simulink model "BenchtopSkinpatch_SingleTone"  (R2016a)
settings: Solver=VariableStepAuto  StartTime=0.0  StopTime=sim_time  RelTol=1e-3
undefined symbols (not defined in the file): Fbit, Fs, Ts, Tsym
libraries: dspsigops x4, commdigbbndpm3 x1
settings Model: Creator=ckilfoyl  LastModifiedBy=ckilfoyl
settings DataIOCC: SaveOutput=off  SignalLogging=off  DSMLogging=off  SaveTime=off  LoggingToFile=on

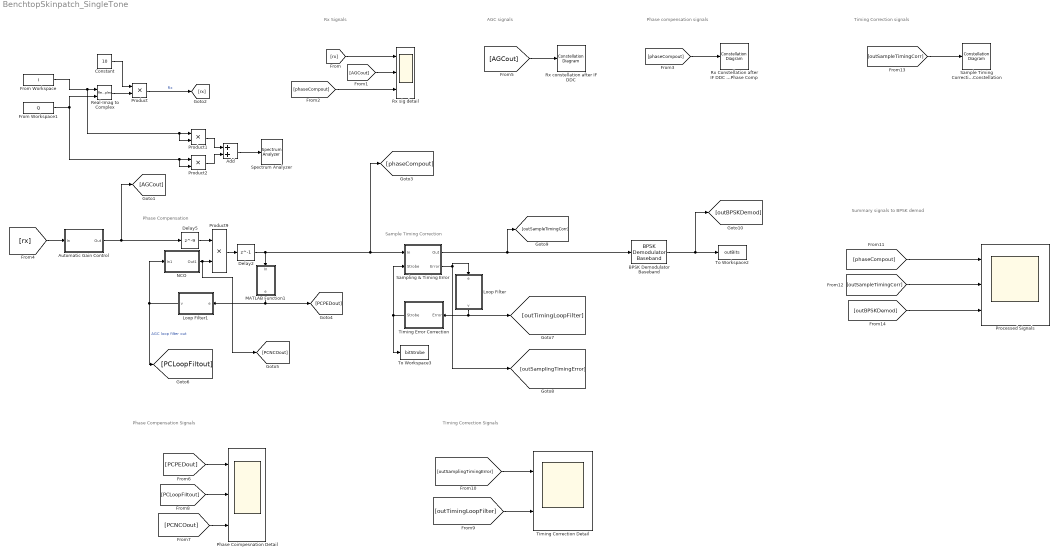
== system BenchtopSkinpatch_SingleTone ==
  note: Phase Compensation Signals
  note: Phase Compensation
  note: Sample Timing Correction
  note: Rx Signals
  note: AGC signals
  note: Phase compensation signals
  note: Timing Correction Signals
  note: Timing Correction signals
  note: Summary signals to BPSK demod
  Add : Sum
  Automatic Gain Control : Subsystem  mask{AGCLoopGain=1, AGCUpperLimit=1000, AGCRef=1}
      mask prompts: AGCLoopGain "Loop Gain"; AGCUpperLimit "Maximum Gain"; AGCRef "Desired Amplitude"
  BPSK Demodulator Baseband : commdigbbndpm3/BPSK Demodulator Baseband  DecType=Hard decision  VarSource=Dialog  Variance=1  Ph=0  outDtype=Inherit via internal rule  derotateFactorWordLen=16  derotateFactorDataTypeStr=Inherit: Same word length as input  derotateFactorLastDataTypeStr=Inherit: Same word length as input
  Constant : Constant  Value=10
  Delay2 : Delay  DelayLength=1  InitialCondition=0
  Delay5 : Delay  DelayLength=9  InitialCondition=0
  From Workspace : FromWorkspace  VariableName=I  OutDataTypeStr=double  SampleTime=Ts  OutputAfterFinalValue=Setting to zero
  From Workspace1 : FromWorkspace  VariableName=Q  OutDataTypeStr=double  SampleTime=Ts  OutputAfterFinalValue=Setting to zero
  Loop Filter : Subsystem  mask{BnTs=.1, zeta=2, N=Fs/Fbit, Kp=0.5, K0=1}
      mask prompts: BnTs "Normalized Loop Bandwidth"; zeta "Damping Factor"; N "Number of Samples/Symbol"; Kp "Phase Detector Gain (Kp)"; K0 "DDS Gain (K0)"
      mask init:
      | % See C.57 to C.61 in Michael Rice's "Digital Communications 
      | % - A Discrete-Time Approach" for details
      | theta = BnTs/(zeta+0.25/zeta)/N;
      | d = 1 + 2*zeta*theta + theta*theta;
      | K1 = 4*zeta*theta/d;
      | K2 = 4*theta*theta/d;
      | K1 = K1/(Kp*K0);
      | K2 = K2/(Kp*K0);
      mask Display: disp('Loop Filter')
  Loop Filter1 : Subsystem  mask{BnTs=.1, zeta=2, N=Fs/Fbit, Kp=2, K0=1}
      mask prompts: BnTs "Normalized Loop Bandwidth"; zeta "Damping Factor"; N "Number of Samples/Symbol"; Kp "Phase Detector Gain (Kp)"; K0 "DDS Gain (K0)"
      mask init: same as BenchtopSkinpatch_SingleTone/Loop Filter
      mask Display: disp('Loop Filter')
  MATLAB Function1 : MATLAB Function  TreatAsAtomicUnit=on
  NCO : Subsystem
  Phase Coimpesnation Detail : Scope  NumInputPorts=3
  Processed Signals : Scope  NumInputPorts=3
  Product : Product
  Product1 : Product
  Product2 : Product
  Product9 : Product  OutDataTypeStr=fixdt(1,16,14)  SaturateOnIntegerOverflow=on  RndMeth=Zero
  Real-Imag to Complex : RealImagToComplex
  Rx Constellation after IF DDC and Phase Comp : ConstellationDiagram
  Rx constellation after IF DDC : ConstellationDiagram
  Rx sig detail : Scope  NumInputPorts=3
  Sample Timing Correction Constellation : ConstellationDiagram
  Sampling & Timing Error : Subsystem
  Spectrum Analyzer : SpectrumAnalyzer
  Timing Correction Detail : Scope  NumInputPorts=2
  Timing Error Correction : Subsystem
  To Workspace2 : ToWorkspace  VariableName=outBits  SaveFormat=Timeseries  SampleTime=-1
  To Workspace3 : ToWorkspace  VariableName=bitStrobe  SaveFormat=Timeseries  SampleTime=-1
  wires:
  [rx] -> Automatic Gain Control/1(In)
  From Workspace/1 -> Product1/2, Product1/1, Real-Imag to Complex/1
  From Workspace1/1 -> Product2/2, Product2/1, Real-Imag to Complex/2
  Product/1 -> [rx]  "Rx"
  Constant/1 -> Product/1
  Sampling & Timing Error/1(Out) -> [outSampleTimingCorr], BPSK Demodulator Baseband/1
  BPSK Demodulator Baseband/1 -> [outBPSKDemod], To Workspace2/1
  Automatic Gain Control/1(Out) -> Delay5/1, [AGCout]
  Delay5/1 -> Product9/1
  Product9/1 -> Delay2/1
  MATLAB Function1/1(e) -> [PCPEDout], Loop Filter1/1(e)
  NCO/1(Out1) -> [PCNCOout], Product9/2
  Loop Filter1/1(v) -> NCO/1(In1), [PCLoopFiltout]  "AGC loop filter out"
  [rx] -> Rx sig detail/1
  [AGCout] -> Rx sig detail/2
  [phaseCompout] -> Rx sig detail/3
  [phaseCompout] -> Rx Constellation after IF DDC and Phase Comp/1
  [AGCout] -> Rx constellation after IF DDC/1
  [PCPEDout] -> Phase Coimpesnation Detail/1
  [PCNCOout] -> Phase Coimpesnation Detail/3
  [PCLoopFiltout] -> Phase Coimpesnation Detail/2
  [outTimingLoopFilter] -> Timing Correction Detail/2
  [outSamplingTimingError] -> Timing Correction Detail/1
  Sampling & Timing Error/2(Error) -> Loop Filter/1(e), [outSamplingTimingError]
  Timing Error Correction/1(Strobe) -> To Workspace3/1, Sampling & Timing Error/2(Strobe)
  Loop Filter/1(v) -> [outTimingLoopFilter], Timing Error Correction/1(Error)
  [phaseCompout] -> Processed Signals/1
  [outSampleTimingCorr] -> Processed Signals/2
  [outSampleTimingCorr] -> Sample Timing Correction Constellation/1
  [outBPSKDemod] -> Processed Signals/3
  Real-Imag to Complex/1 -> Product/2
  Delay2/1 -> [phaseCompout], Sampling & Timing Error/1(In), MATLAB Function1/1(In)
  Product1/1 -> Add/1
  Product2/1 -> Add/2
  Add/1 -> Spectrum Analyzer/1

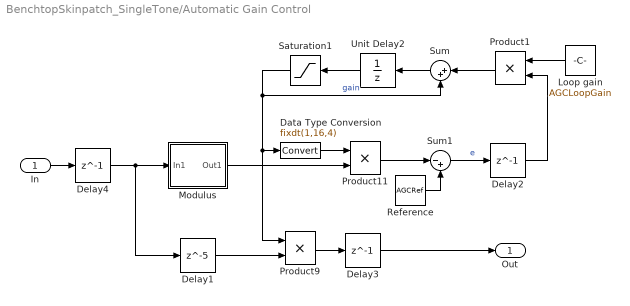
== system BenchtopSkinpatch_SingleTone/Automatic Gain Control ==
  In : Inport
  Data Type Conversion : DataTypeConversion  OutDataTypeStr=fixdt(1,16,4)  SaturateOnIntegerOverflow=on
  Delay1 : Delay  DelayLength=5  InitialCondition=0
  Delay2 : Delay  DelayLength=1  InitialCondition=0
  Delay3 : Delay  DelayLength=1  InitialCondition=0
  Delay4 : Delay  DelayLength=1  InitialCondition=0
  Loop gain : Constant  Value=AGCLoopGain  OutDataTypeStr=fixdt(1,16,10)  SampleTime=Ts
  Modulus : Subsystem
  Product1 : Product  OutDataTypeStr=fixdt(1,16,10)  RndMeth=Zero
  Product11 : Product  OutDataTypeStr=fixdt(1,16,10)  RndMeth=Zero
  Product9 : Product  OutDataTypeStr=fixdt(1,16,14)  SaturateOnIntegerOverflow=on  RndMeth=Zero
  Reference : Constant  Value=AGCRef  OutDataTypeStr=fixdt(1,16,10)  SampleTime=Ts
  Saturation1 : Saturate  UpperLimit=AGCUpperLimit  LowerLimit=1e-5
  Sum : Sum  Inputs=|++  OutDataTypeStr=fixdt(1,23,10)  SaturateOnIntegerOverflow=on
  Sum1 : Sum  Inputs=|-+  OutDataTypeStr=Inherit: Same as first input
  Unit Delay2 : UnitDelay  SampleTime=-1
  Out : Outport  PortDimensions=1
  wires:
  Saturation1/1 -> Sum/2, Product9/1, Data Type Conversion/1  "gain"
  Loop gain/1 -> Product1/1
  Product1/1 -> Sum/1
  Modulus/1(Out1) -> Product11/2
  Delay4/1 -> Modulus/1(In1), Delay1/1
  Unit Delay2/1 -> Saturation1/1
  Delay2/1 -> Product1/2
  Delay3/1 -> Out/1
  Delay1/1 -> Product9/2
  Product9/1 -> Delay3/1
  Sum1/1 -> Delay2/1  "e"
  Sum/1 -> Unit Delay2/1
  Reference/1 -> Sum1/2
  Data Type Conversion/1 -> Product11/1
  Product11/1 -> Sum1/1
  In/1 -> Delay4/1

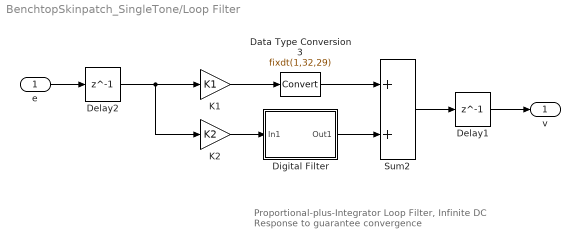
== system BenchtopSkinpatch_SingleTone/Loop Filter ==
  note: Proportional-plus-Integrator Loop Filter,
      | Infinite DC Response to guarantee convergence
  e : Inport
  Data Type Conversion3 : DataTypeConversion  OutDataTypeStr=fixdt(1,32,29)
  Delay1 : Delay  DelayLength=1  InitialCondition=0
  Delay2 : Delay  DelayLength=1  InitialCondition=0
  Digital Filter : Subsystem
  K1 : Gain  Gain=K1
  K2 : Gain  Gain=K2
  Sum2 : Sum  OutDataTypeStr=fixdt(1,22,19)  SaturateOnIntegerOverflow=on  InputSameDT=on
  v : Outport
  wires:
  Delay1/1 -> v/1
  Digital Filter/1(Out1) -> Sum2/2
  Sum2/1 -> Delay1/1
  K2/1 -> Digital Filter/1(In1)
  Data Type Conversion3/1 -> Sum2/1
  Delay2/1 -> K2/1, K1/1
  e/1 -> Delay2/1
  K1/1 -> Data Type Conversion3/1

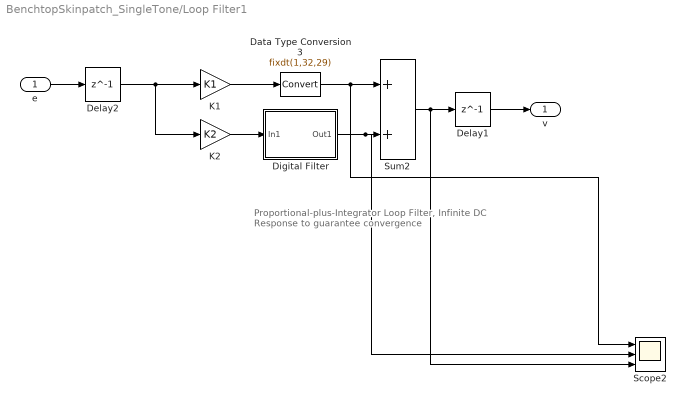
== system BenchtopSkinpatch_SingleTone/Loop Filter1 ==
  note: Proportional-plus-Integrator Loop Filter,
      | Infinite DC Response to guarantee convergence
  e : Inport
  Data Type Conversion3 : DataTypeConversion  OutDataTypeStr=fixdt(1,32,29)
  Delay1 : Delay  DelayLength=1  InitialCondition=0
  Delay2 : Delay  DelayLength=1  InitialCondition=0
  Digital Filter : Subsystem
  K1 : Gain  Gain=K1
  K2 : Gain  Gain=K2
  Scope2 : Scope  NumInputPorts=3
  Sum2 : Sum  OutDataTypeStr=fixdt(1,22,19)  SaturateOnIntegerOverflow=on  InputSameDT=on
  v : Outport
  wires:
  Delay1/1 -> v/1
  Digital Filter/1(Out1) -> Scope2/2, Sum2/2
  Sum2/1 -> Scope2/3, Delay1/1
  K2/1 -> Digital Filter/1(In1)
  Data Type Conversion3/1 -> Scope2/1, Sum2/1
  Delay2/1 -> K2/1, K1/1
  e/1 -> Delay2/1
  K1/1 -> Data Type Conversion3/1

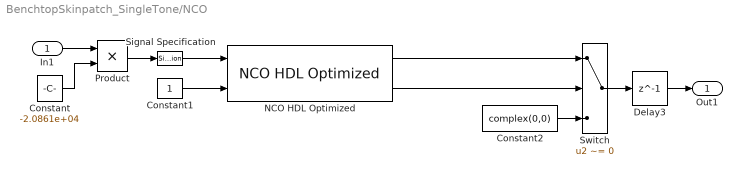
== system BenchtopSkinpatch_SingleTone/NCO ==
  In1 : Inport
  Constant : Constant  Value=-2.0861e+04  OutDataTypeStr=int16  SampleTime=Ts
  Constant1 : Constant  OutDataTypeStr=boolean  SampleTime=Ts
  Constant2 : Constant  Value=complex(0,0)  OutDataTypeStr=fixdt(1,10,8)  SampleTime=Ts
  Delay3 : Delay  DelayLength=1  InitialCondition=0
  NCO HDL Optimized : dspsigops/NCO HDL Optimized  PhaseIncrementSource=Input port  PhaseIncrement=100  PhaseOffsetSource=Property  PhaseOffset=0  DitherSource=None  NumDitherBits=1  PhaseQuantization=on  NumQuantizerAccumulatorBits=16  LUTCompress=on  ResetAction=off  ValidInputPort=on  Waveform=Complex exponential  PhasePort=off  AccumulatorWL=17  OutputDataType=Binary point scaling  OutputWL=10  OutputFL=8  SimulateUsing=Code generation
  Product : Product  OutDataTypeStr=int16
  Signal Specification : SignalSpecification  Dimensions=1
  Switch : Switch  Criteria=u2 ~= 0
  Out1 : Outport
  wires:
  Delay3/1 -> Out1/1
  Constant2/1 -> Switch/3
  NCO HDL Optimized/2 -> Switch/2
  Constant1/1 -> NCO HDL Optimized/2
  NCO HDL Optimized/1 -> Switch/1
  Signal Specification/1 -> NCO HDL Optimized/1
  Switch/1 -> Delay3/1
  Product/1 -> Signal Specification/1
  Constant/1 -> Product/2
  In1/1 -> Product/1

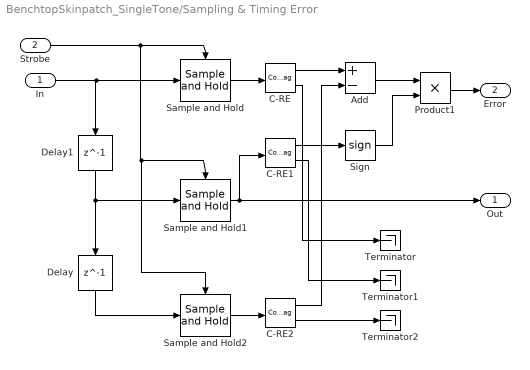
== system BenchtopSkinpatch_SingleTone/Sampling & Timing Error ==
  In : Inport
  Strobe : Inport  Port=2
  Add : Sum  Inputs=+-
  C-RE : ComplexToRealImag
  C-RE1 : ComplexToRealImag
  C-RE2 : ComplexToRealImag
  Delay : Delay  DelayLength=1  InitialCondition=0
  Delay1 : Delay  DelayLength=1  InitialCondition=0
  Product1 : Product
  Sample and Hold : dspsigops/Sample and Hold  trig=Rising edge  initCond=0  latchinput=off
  Sample and Hold1 : dspsigops/Sample and Hold  trig=Rising edge  initCond=0  latchinput=off
  Sample and Hold2 : dspsigops/Sample and Hold  trig=Rising edge  initCond=0  latchinput=off
  Sign : Signum
  Terminator : Terminator
  Terminator1 : Terminator
  Terminator2 : Terminator
  Out : Outport
  Error : Outport  Port=2
  wires:
  Delay1/1 -> Sample and Hold1/1, Delay/1
  Delay/1 -> Sample and Hold2/1
  Strobe/1 -> Sample and Hold2/Trigger, Sample and Hold1/Trigger, Sample and Hold/Trigger
  Sign/1 -> Product1/2
  Add/1 -> Product1/1
  Sample and Hold1/1 -> Out/1, C-RE1/1
  In/1 -> Delay1/1, Sample and Hold/1
  Product1/1 -> Error/1
  Sample and Hold/1 -> C-RE/1
  C-RE/1 -> Add/1
  C-RE2/1 -> Add/2
  Sample and Hold2/1 -> C-RE2/1
  C-RE1/1 -> Sign/1
  C-RE2/2 -> Terminator2/1
  C-RE1/2 -> Terminator1/1
  C-RE/2 -> Terminator/1

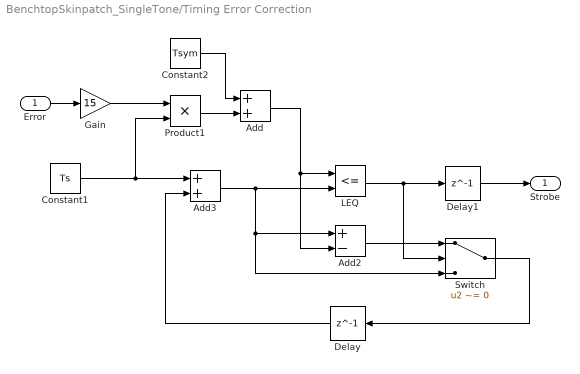
== system BenchtopSkinpatch_SingleTone/Timing Error Correction ==
  Error : Inport
  Add : Sum
  Add2 : Sum  Inputs=+-
  Add3 : Sum
  Constant1 : Constant  Value=Ts  SampleTime=-1
  Constant2 : Constant  Value=Tsym  SampleTime=-1
  Delay : Delay  DelayLength=1  InitialCondition=0
  Delay1 : Delay  DelayLength=1  InitialCondition=0
  Gain : Gain  Gain=15
  LEQ : RelationalOperator  Operator=<=  OutDataTypeStr=boolean
  Product1 : Product
  Switch : Switch  Criteria=u2 ~= 0
  Strobe : Outport
  wires:
  Constant1/1 -> Product1/2, Add3/1
  Add/1 -> Add2/2, LEQ/1
  Add2/1 -> Switch/1
  Error/1 -> Gain/1
  Constant2/1 -> Add/1
  Add3/1 -> Switch/3, Add2/1, LEQ/2
  Switch/1 -> Delay/1
  Product1/1 -> Add/2
  LEQ/1 -> Delay1/1, Switch/2
  Delay/1 -> Add3/2
  Delay1/1 -> Strobe/1
  Gain/1 -> Product1/1

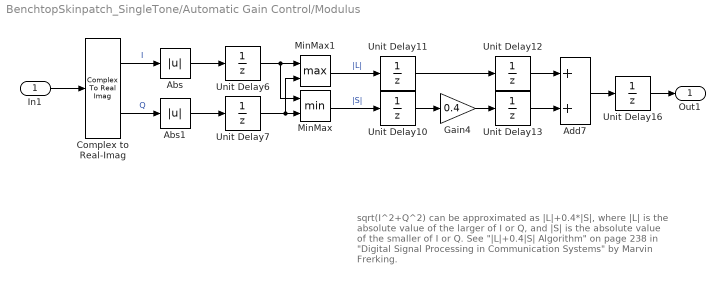
== system BenchtopSkinpatch_SingleTone/Automatic Gain Control/Modulus ==
  note: sqrt(I^2+Q^2) can be approximated as |L|+0.4*|S|,
      | where |L| is the absolute value of the larger of I or Q,
      | and |S| is the absolute value of the smaller of I or Q.
      |
      | See "|L|+0.4|S| Algorithm" on page 238 in "Digital Signal
      | Processing in Communication Systems" by Marvin Frerking.
  In1 : Inport
  Abs : Abs
  Abs1 : Abs
  Add7 : Sum
  Complex to Real-Imag : ComplexToRealImag
  Gain4 : Gain  Gain=0.4  OutDataTypeStr=fixdt(1,16,15)
  MinMax : MinMax  Inputs=2
  MinMax1 : MinMax  Function=max  Inputs=2
  Unit Delay{6..7,10..13,16} (7 alike) : UnitDelay  SampleTime=-1
  Out1 : Outport
  wires:
  In1/1 -> Complex to Real-Imag/1
  Unit Delay7/1 -> MinMax/2, MinMax1/2
  Unit Delay6/1 -> MinMax1/1, MinMax/1
  MinMax/1 -> Unit Delay10/1  "|S|"
  Gain4/1 -> Unit Delay13/1
  Unit Delay13/1 -> Add7/2
  MinMax1/1 -> Unit Delay11/1  "|L|"
  Complex to Real-Imag/2 -> Abs1/1  "Q"
  Complex to Real-Imag/1 -> Abs/1  "I"
  Abs/1 -> Unit Delay6/1
  Add7/1 -> Unit Delay16/1
  Abs1/1 -> Unit Delay7/1
  Unit Delay12/1 -> Add7/1
  Unit Delay10/1 -> Gain4/1
  Unit Delay16/1 -> Out1/1
  Unit Delay11/1 -> Unit Delay12/1

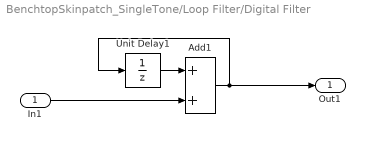
== system BenchtopSkinpatch_SingleTone/Loop Filter/Digital Filter ==
  In1 : Inport
  Add1 : Sum  OutDataTypeStr=fixdt(1,32,29)
  Unit Delay1 : UnitDelay  SampleTime=-1
  Out1 : Outport
  wires:
  Unit Delay1/1 -> Add1/1
  Add1/1 -> Out1/1, Unit Delay1/1
  In1/1 -> Add1/2

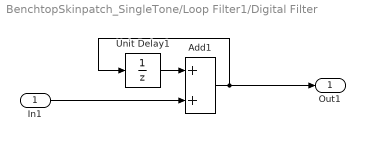
== system BenchtopSkinpatch_SingleTone/Loop Filter1/Digital Filter ==
  In1 : Inport
  Add1 : Sum  OutDataTypeStr=fixdt(1,32,29)
  Unit Delay1 : UnitDelay  SampleTime=-1
  Out1 : Outport
  wires:
  Unit Delay1/1 -> Add1/1
  Add1/1 -> Out1/1, Unit Delay1/1
  In1/1 -> Add1/2

== matlab function BenchtopSkinpatch_SingleTone/MATLAB Function1 ==
  data: In input; e output
function e  = PED(In)
% Input:
%   In - Input samples, oversampled by two
% Output:
%   e - Phase error
% PED implements 
% e = sign(imag(In)).*imag(In) - sign(real(In)).*real(In);

%#codegen

% OP1 = real(In);
% OP2 = imag(In);
% 
% Real = OP1;
% Imag = OP2;
% 
% if(bitget(Real,16)==true)%real is negative
%     OP1 = fi(-Imag,1,16,14);
% end
% if(bitget(Real,16)==false)%real is positive
%     OP1 = fi(Imag,1,16,14);
% end
% 
% e = fi(OP1,1,16,14);

OP1 = real(In);
OP2 = imag(In);

Real = OP1;
Imag = OP2;
OP3 = OP1;

if (bitget(Real,16)==false)%real part positive
    OP1 = fi((1-Real),1,16,14);
    OP2 = fi(Imag,1,16,14);
end
if (bitget(Real,16)==true)%real part negative
    OP1 = fi(-(1+Real),1,16,14);
    OP2 = fi(-Imag,1,16,14);
end

if(bitget(Imag,16)==false)%imag part positive
    OP3 = fi(OP2 + OP1,1,16,14);
end
if(bitget(Imag,16)==true)%imag part negative
    OP3 = fi(OP2 - OP1,1,16,14);
end

e= fi(OP3,1,16,14);
